simulink model "example_battery"  (R2018b)
settings: Solver=VariableStepAuto  StartTime=0.0  StopTime=24*3600  RelTol=1e-3
undefined symbols (not defined in the file): sigbuilder_block
libraries: carnot x2
settings Model: Creator=drhf  LastModifiedBy=drhf
settings SFSimCC: SimUseLocalCustomCode=off
settings RTWCC: RTWUseLocalCustomCode=off
settings CodeAppCC: StateflowObjectComments=on

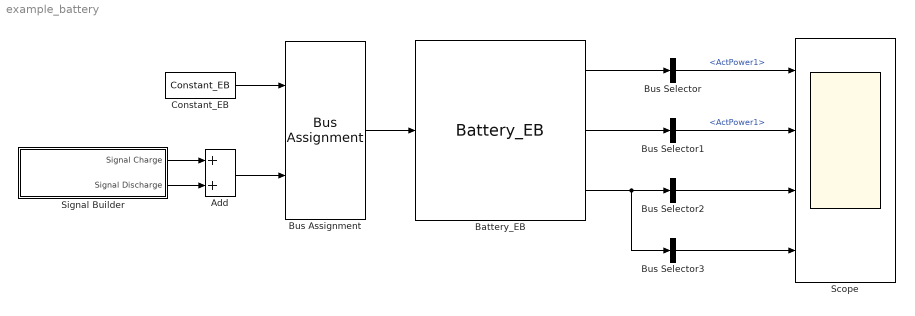
== system example_battery ==
  Add : Sum
  Battery_EB : carnot/Storage/Electric/Battery_EB  cap_kWh=10  eta_ch=0.95  eta_dis=0.95  cap0=0.5  SOC_max=1  SOC_min=0  Pmax=3000  Pmin=-3000  P_standby=0
      settings: SourceProductName=Carnot
  Bus Assignment : BusAssignment  AssignedSignals=ActPower1
  Bus Selector : BusSelector  OutputSignals=ActPower1
  Bus Selector1 : BusSelector  OutputSignals=ActPower1
  Bus Selector2 : BusSelector  OutputSignals=Psat,Peff,Pcharge_DC,Pdischarge_DC  OutputAsBus=on
  Bus Selector3 : BusSelector  OutputSignals=Pover,Punder  OutputAsBus=on
  Constant_EB : carnot/Source/Simple/Constant_EB  eID=Power only  f=50  v1=230  p1=0  pf1=1  v2=230  p2=0  pf2=1  v3=230  p3=0  pf3=1
      settings: SourceProductName=Carnot
  Scope : Scope  NumInputPorts=4
  Signal Builder : Subsystem  Tag=STV Subsys  LoadFcn=sigbuilder_block('load');  StartFcn=sigbuilder_block('start');  StopFcn=sigbuilder_block('stop');  ClipboardFcn=sigbuilder_block('clipboard');  mask(Sigbuilder block){tuvar=[0:10]}
      mask help: Simulink:masks:SigbuilderBlock_MD
      mask init:
      | if ~strcmp(get_param(bdroot(gcbh),'SimulationStatus'),'stopped') tuvar = sigbuilder_block('maskInit'); end
      settings: CopyFcn=sigbuilder_block('copy');  DeleteFcn=sigbuilder_block('delete');  ModelCloseFcn=sigbuilder_block('modelClose');  PreSaveFcn=sigbuilder_block('preSave');  PauseFcn=sigbuilder_block('pause');  ContinueFcn=sigbuilder_block('continue');  NameChangeFcn=sigbuilder_block('namechange');  OpenFcn=sigbuilder_block('open',[437.25 136.5 681.75 462.75 ]);  CloseFcn=sigbuilder_block('close');
      mask Display: plot(0, 0, 100, 100,[2, 2, 32, 32, 2], [68, 8, 8, 68, 68],[32, 2], [38, 38], [32, 19, 2],[53, 60, 44], [32, 17, 17, 2],[16, 16, 31, 31]);txt = getActiveGroup(gcbh);text(2, 100, txt,'verticalAlignment', 'top');
  wires:
  Bus Assignment/1 -> Battery_EB/1
  Add/1 -> Bus Assignment/2
  Signal Builder/1(Signal Charge) -> Add/1
  Signal Builder/2(Signal Discharge) -> Add/2
  Battery_EB/1 -> Bus Selector/1
  Battery_EB/2 -> Bus Selector1/1
  Battery_EB/3 -> Bus Selector3/1, Bus Selector2/1
  Bus Selector/1 -> Scope/1  "<ActPower1>"
  Bus Selector1/1 -> Scope/2  "<ActPower1>"
  Bus Selector2/1 -> Scope/3
  Bus Selector3/1 -> Scope/4
  Constant_EB/1 -> Bus Assignment/1

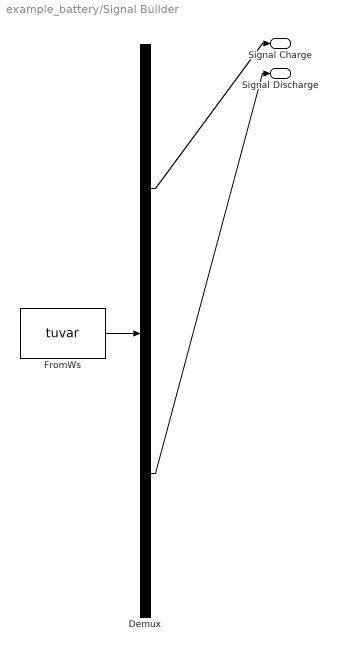
== system example_battery/Signal Builder ==
  Demux : Demux  Tag=STV Demux  Outputs=2
  FromWs : FromWorkspace  Tag=STV FromWs  VariableName=tuvar  SampleTime=0
      SigBuilderData=|
      | common.afterFinalStr = 'Extrapolate'
      | common.sampleTime = 0
      | dataSet.timeRange = [0 86400]
      | dataSet.name = 'Group 1'
      | sbobj.Groups.Name = 'Group 1'
      | sbobj.Groups.Signals(1).Name = 'Signal Charge'
      | sbobj.Groups.Signals(1).XData = [0 7200 7200 43200 43200 86400]
      | sbobj.Groups.Signals(1).YData = [0 0 1000 1000 0 0]
      | sbobj.Groups.Signals(2).Name = 'Signal Discharge'
      | sbobj.Groups.Signals(2).XData = [0 46800 46800 82800 82800 86400]
      | sbobj.Groups.Signals(2).YData = [0 0 -1000 -1000 0 0]
      | sbobj.Groups.TimeRange = [0 86400]
  Signal Charge : Outport  Tag=STV Outport
  Signal Discharge : Outport  Tag=STV Outport  Port=2
  wires:
  FromWs/1 -> Demux/1
  Demux/1 -> Signal Charge/1
  Demux/2 -> Signal Discharge/1
